simulink model "ERMF_main"  (R2015a)
settings: Solver=ode45  StartTime=0.0  StopTime=10.0  RelTol=1e-3
undefined symbols (not defined in the file or in its folder): EOM
libraries: aerolibutil x4, AERO_lib x1, ATM_lib x1, aerolib6dof2 x1, MOT_lib x1
settings Model: Creator=Andrew  LastModifiedBy=Andrew

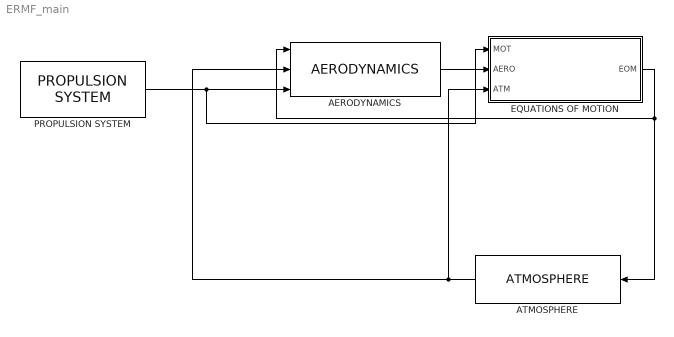
== system ERMF_main ==
  AERODYNAMICS : AERO_lib/AERODYNAMICS
  ATMOSPHERE : ATM_lib/ATMOSPHERE
  EQUATIONS OF MOTION : Subsystem  AncestorBlock=EOM_lib/EQUATIONS OF MOTION
  PROPULSION SYSTEM : MOT_lib/PROPULSION SYSTEM
  wires:
  ATMOSPHERE/1 -> EQUATIONS OF MOTION/3(ATM), AERODYNAMICS/2
  AERODYNAMICS/1 -> EQUATIONS OF MOTION/2(AERO)
  PROPULSION SYSTEM/1 -> EQUATIONS OF MOTION/1(MOT), AERODYNAMICS/3
  EQUATIONS OF MOTION/1(EOM) -> ATMOSPHERE/1, AERODYNAMICS/1

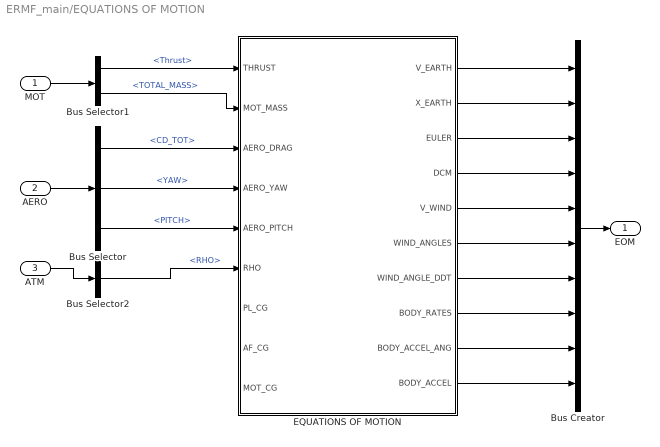
== system ERMF_main/EQUATIONS OF MOTION ==
  MOT : Inport
  AERO : Inport  Port=2
  ATM : Inport  Port=3
  Bus Creator : BusCreator  Inputs=10
  Bus Selector : BusSelector  OutputSignals=AERO_PROP.CD_TOT,VEHICLE.AIRFRAME.YAW,VEHICLE.AIRFRAME.PITCH
  Bus Selector1 : BusSelector  OutputSignals=Thrust,TOTAL_MASS
  Bus Selector2 : BusSelector  OutputSignals=RHO
  EQUATIONS OF MOTION : Subsystem
  EOM : Outport
  wires:
  AERO/1 -> Bus Selector/1
  Bus Selector/1 -> EQUATIONS OF MOTION/3(AERO_DRAG)  "<CD_TOT>"
  Bus Selector/3 -> EQUATIONS OF MOTION/5(AERO_PITCH)  "<PITCH>"
  Bus Selector/2 -> EQUATIONS OF MOTION/4(AERO_YAW)  "<YAW>"
  MOT/1 -> Bus Selector1/1
  Bus Selector1/1 -> EQUATIONS OF MOTION/1(THRUST)  "<Thrust>"
  Bus Selector1/2 -> EQUATIONS OF MOTION/2(MOT_MASS)  "<TOTAL_MASS>"
  ATM/1 -> Bus Selector2/1
  Bus Selector2/1 -> EQUATIONS OF MOTION/6(RHO)  "<RHO>"
  Bus Creator/1 -> EOM/1
  EQUATIONS OF MOTION/4(DCM) -> Bus Creator/4
  EQUATIONS OF MOTION/5(V_WIND) -> Bus Creator/5
  EQUATIONS OF MOTION/2(X_EARTH) -> Bus Creator/2
  EQUATIONS OF MOTION/3(EULER) -> Bus Creator/3
  EQUATIONS OF MOTION/1(V_EARTH) -> Bus Creator/1
  EQUATIONS OF MOTION/9(BODY_ACCEL_ANG) -> Bus Creator/9
  EQUATIONS OF MOTION/10(BODY_ACCEL) -> Bus Creator/10
  EQUATIONS OF MOTION/6(WIND_ANGLES) -> Bus Creator/6
  EQUATIONS OF MOTION/8(BODY_RATES) -> Bus Creator/8
  EQUATIONS OF MOTION/7(WIND_ANGLE_DDT) -> Bus Creator/7

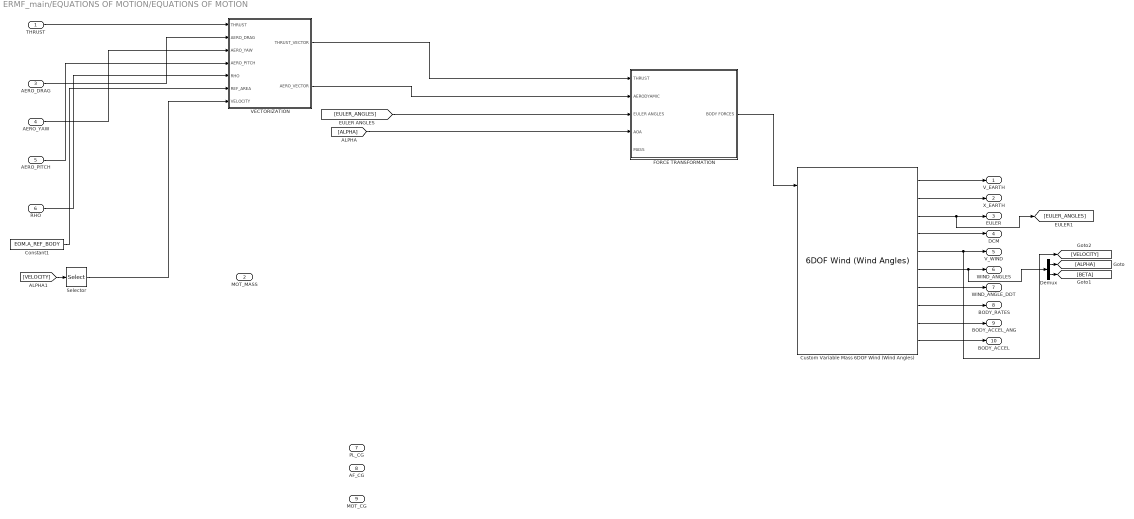
== system ERMF_main/EQUATIONS OF MOTION/EQUATIONS OF MOTION ==
  THRUST : Inport
  MOT_MASS : Inport  Port=2
  AERO_DRAG : Inport  Port=3
  AERO_YAW : Inport  Port=4
  AERO_PITCH : Inport  Port=5
  RHO : Inport  Port=6
  PL_CG : Inport  Port=7
  AF_CG : Inport  Port=8
  MOT_CG : Inport  Port=9
  Constant1 : Constant  Value=EOM.A_REF_BODY
  Custom Variable Mass 6DOF Wind (Wind Angles) : aerolib6dof2/6DOF Wind (Wind Angles)  units=Metric (MKS)  mtype=Custom Variable  rep=Wind Angles  xme_0=[0 0 0]  Vm_0=[0 0 0]  wind_0=[0 0 0]  pm_0=[0 0 0]  mass_0=1.0  mass_e=0.5  mass_f=2.0  inertia=eye(3)  inertia_e=eye(3)  inertia_f=2*eye(3)  vre_flag=off
  Demux : Demux  Outputs=2
  FORCE TRANSFORMATION : Subsystem
  Selector : Selector  InputPortWidth=3  Indices=[1]
  VECTORIZATION : Subsystem
  V_EARTH : Outport
  X_EARTH : Outport  Port=2
  EULER : Outport  Port=3
  DCM : Outport  Port=4
  V_WIND : Outport  Port=5
  WIND_ANGLES : Outport  Port=6
  WIND_ANGLE_DDT : Outport  Port=7
  BODY_RATES : Outport  Port=8
  BODY_ACCEL_ANG : Outport  Port=9
  BODY_ACCEL : Outport  Port=10
  wires:
  [EULER_ANGLES] -> FORCE TRANSFORMATION/3(EULER ANGLES)
  FORCE TRANSFORMATION/1(BODY FORCES) -> Custom Variable Mass 6DOF Wind (Wind Angles)/1
  [ALPHA] -> FORCE TRANSFORMATION/4(AOA)
  Demux/1 -> [ALPHA]
  Demux/2 -> [BETA]
  Custom Variable Mass 6DOF Wind (Wind Angles)/1 -> V_EARTH/1
  Custom Variable Mass 6DOF Wind (Wind Angles)/2 -> X_EARTH/1
  Custom Variable Mass 6DOF Wind (Wind Angles)/3 -> [EULER_ANGLES], EULER/1
  Custom Variable Mass 6DOF Wind (Wind Angles)/4 -> DCM/1
  Custom Variable Mass 6DOF Wind (Wind Angles)/5 -> [VELOCITY], V_WIND/1
  Custom Variable Mass 6DOF Wind (Wind Angles)/6 -> Demux/1, WIND_ANGLES/1
  Custom Variable Mass 6DOF Wind (Wind Angles)/7 -> WIND_ANGLE_DDT/1
  Custom Variable Mass 6DOF Wind (Wind Angles)/8 -> BODY_RATES/1
  Custom Variable Mass 6DOF Wind (Wind Angles)/9 -> BODY_ACCEL_ANG/1
  Custom Variable Mass 6DOF Wind (Wind Angles)/10 -> BODY_ACCEL/1
  THRUST/1 -> VECTORIZATION/1(THRUST)
  AERO_DRAG/1 -> VECTORIZATION/2(AERO_DRAG)
  AERO_YAW/1 -> VECTORIZATION/3(AERO_YAW)
  AERO_PITCH/1 -> VECTORIZATION/4(AERO_PITCH)
  RHO/1 -> VECTORIZATION/5(RHO)
  Constant1/1 -> VECTORIZATION/6(REF_AREA)
  VECTORIZATION/1(THRUST_VECTOR) -> FORCE TRANSFORMATION/1(THRUST)
  VECTORIZATION/2(AERO_VECTOR) -> FORCE TRANSFORMATION/2(AERODYAMIC)
  [VELOCITY] -> Selector/1
  Selector/1 -> VECTORIZATION/7(VELOCITY)

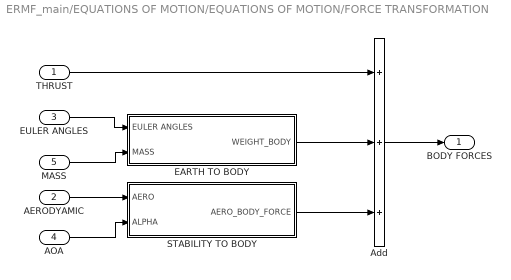
== system ERMF_main/EQUATIONS OF MOTION/EQUATIONS OF MOTION/FORCE TRANSFORMATION ==
  THRUST : Inport
  AERODYAMIC : Inport  Port=2
  EULER ANGLES : Inport  Port=3
  AOA : Inport  Port=4
  MASS : Inport  Port=5
  Add : Sum  Inputs=+++
  EARTH TO BODY : Subsystem
  STABILITY TO BODY : Subsystem
  BODY FORCES : Outport
  wires:
  AOA/1 -> STABILITY TO BODY/2(ALPHA)
  Add/1 -> BODY FORCES/1
  THRUST/1 -> Add/1
  STABILITY TO BODY/1(AERO_BODY_FORCE) -> Add/3
  AERODYAMIC/1 -> STABILITY TO BODY/1(AERO)
  EARTH TO BODY/1(WEIGHT_BODY) -> Add/2
  MASS/1 -> EARTH TO BODY/2(MASS)
  EULER ANGLES/1 -> EARTH TO BODY/1(EULER ANGLES)

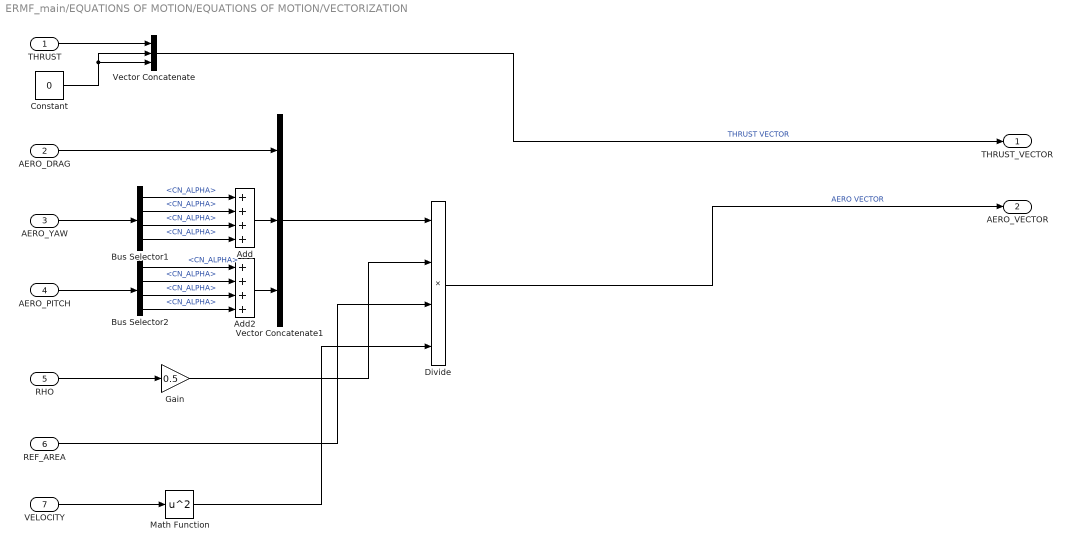
== system ERMF_main/EQUATIONS OF MOTION/EQUATIONS OF MOTION/VECTORIZATION ==
  THRUST : Inport
  AERO_DRAG : Inport  Port=2
  AERO_YAW : Inport  Port=3
  AERO_PITCH : Inport  Port=4
  RHO : Inport  Port=5
  REF_AREA : Inport  Port=6
  VELOCITY : Inport  Port=7
  Add : Sum  Inputs=++++
  Add2 : Sum  Inputs=++++
  Bus Selector1 : BusSelector  OutputSignals=NC.CN_ALPHA,AF_1.CN_ALPHA,AF_2.CN_ALPHA,FIN.CN_ALPHA
  Bus Selector2 : BusSelector  OutputSignals=NC.CN_ALPHA,AF_1.CN_ALPHA,AF_2.CN_ALPHA,FIN.CN_ALPHA
  Constant : Constant  Value=0
  Divide : Product  Inputs=****
  Gain : Gain  Gain=0.5
  Math Function : Math  Operator=square  SaturateOnIntegerOverflow=on
  Vector Concatenate : Concatenate  NumInputs=3
  Vector Concatenate1 : Concatenate  NumInputs=3
  THRUST_VECTOR : Outport
  AERO_VECTOR : Outport  Port=2
  wires:
  Bus Selector2/2 -> Add2/2  "<CN_ALPHA>"
  Bus Selector2/3 -> Add2/3  "<CN_ALPHA>"
  Divide/1 -> AERO_VECTOR/1  "AERO VECTOR"
  THRUST/1 -> Vector Concatenate/1
  Gain/1 -> Divide/2
  Math Function/1 -> Divide/4
  AERO_DRAG/1 -> Vector Concatenate1/1
  AERO_PITCH/1 -> Bus Selector2/1
  AERO_YAW/1 -> Bus Selector1/1
  Vector Concatenate1/1 -> Divide/1
  VELOCITY/1 -> Math Function/1
  Add/1 -> Vector Concatenate1/2
  REF_AREA/1 -> Divide/3
  Bus Selector1/3 -> Add/3  "<CN_ALPHA>"
  Bus Selector2/1 -> Add2/1  "<CN_ALPHA>"
  Add2/1 -> Vector Concatenate1/3
  Bus Selector2/4 -> Add2/4  "<CN_ALPHA>"
  Bus Selector1/4 -> Add/4  "<CN_ALPHA>"
  Bus Selector1/2 -> Add/2  "<CN_ALPHA>"
  Bus Selector1/1 -> Add/1  "<CN_ALPHA>"
  Vector Concatenate/1 -> THRUST_VECTOR/1  "THRUST VECTOR"
  RHO/1 -> Gain/1
  Constant/1 -> Vector Concatenate/2, Vector Concatenate/3

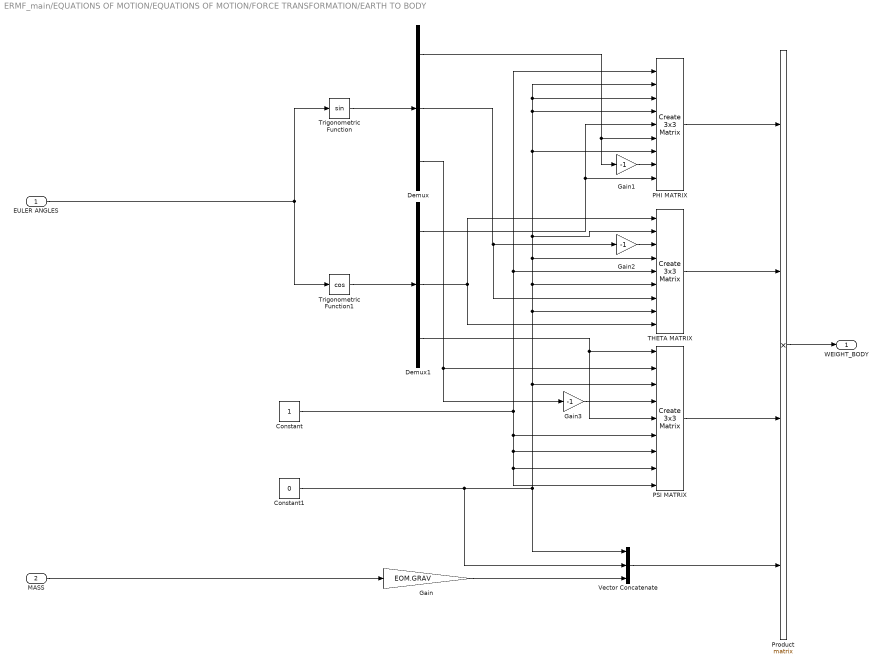
== system ERMF_main/EQUATIONS OF MOTION/EQUATIONS OF MOTION/FORCE TRANSFORMATION/EARTH TO BODY ==
  EULER ANGLES : Inport
  MASS : Inport  Port=2
  Constant : Constant
  Constant1 : Constant  Value=0
  Demux : Demux  Outputs=3
  Demux1 : Demux  Outputs=3
  Gain : Gain  Gain=EOM.GRAV
  Gain1 : Gain  Gain=-1
  Gain2 : Gain  Gain=-1
  Gain3 : Gain  Gain=-1
  "PHI MATRIX " : aerolibutil/Create 3x3 Matrix
  PSI MATRIX : aerolibutil/Create 3x3 Matrix
  Product : Product  Inputs=4  Multiplication=Matrix(*)
  THETA MATRIX : aerolibutil/Create 3x3 Matrix
  Trigonometric Function : Trigonometry
  Trigonometric Function1 : Trigonometry  Operator=cos
  Vector Concatenate : Concatenate  NumInputs=3
  WEIGHT_BODY : Outport
  wires:
  Constant/1 -> THETA MATRIX/5, "PHI MATRIX "/1, PSI MATRIX/6, PSI MATRIX/9, PSI MATRIX/8, PSI MATRIX/7
  Gain1/1 -> "PHI MATRIX "/8
  Gain2/1 -> THETA MATRIX/3
  EULER ANGLES/1 -> Trigonometric Function1/1, Trigonometric Function/1
  Demux1/2 -> THETA MATRIX/9, THETA MATRIX/1
  Demux/2 -> Gain2/1, THETA MATRIX/7
  Trigonometric Function/1 -> Demux/1
  Demux1/1 -> "PHI MATRIX "/9, "PHI MATRIX "/5
  Trigonometric Function1/1 -> Demux1/1
  Constant1/1 -> "PHI MATRIX "/2, "PHI MATRIX "/3, "PHI MATRIX "/4, "PHI MATRIX "/7, THETA MATRIX/2, THETA MATRIX/4, THETA MATRIX/6, THETA MATRIX/8, PSI MATRIX/3, Vector Concatenate/1, Vector Concatenate/2
  Gain/1 -> Vector Concatenate/3
  Demux/1 -> "PHI MATRIX "/6, Gain1/1
  MASS/1 -> Gain/1
  "PHI MATRIX "/1 -> Product/1
  THETA MATRIX/1 -> Product/2
  PSI MATRIX/1 -> Product/3
  Vector Concatenate/1 -> Product/4
  Demux1/3 -> PSI MATRIX/1, PSI MATRIX/5
  Demux/3 -> Gain3/1, PSI MATRIX/2
  Gain3/1 -> PSI MATRIX/4
  Product/1 -> WEIGHT_BODY/1

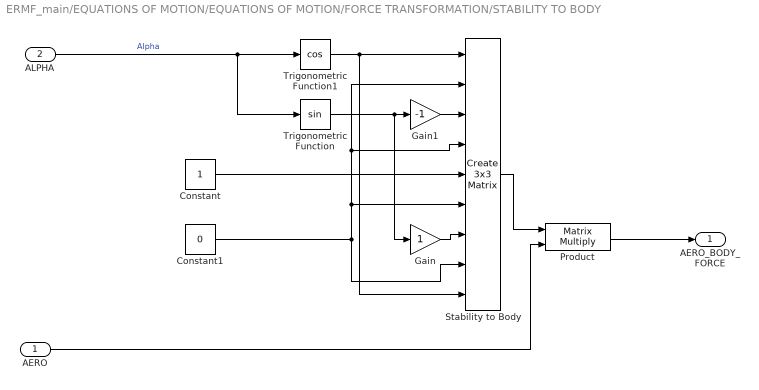
== system ERMF_main/EQUATIONS OF MOTION/EQUATIONS OF MOTION/FORCE TRANSFORMATION/STABILITY TO BODY ==
  AERO : Inport
  ALPHA : Inport  Port=2
  Constant : Constant
  Constant1 : Constant  Value=0
  Gain : Gain
  Gain1 : Gain  Gain=-1
  Product : Product  Multiplication=Matrix(*)
  Stability to Body : aerolibutil/Create 3x3 Matrix
  Trigonometric Function : Trigonometry
  Trigonometric Function1 : Trigonometry  Operator=cos
  AERO_BODY_FORCE : Outport
  wires:
  ALPHA/1 -> Trigonometric Function1/1, Trigonometric Function/1  "Alpha"
  Stability to Body/1 -> Product/1
  Constant/1 -> Stability to Body/5
  Trigonometric Function/1 -> Gain1/1, Gain/1
  Gain1/1 -> Stability to Body/3
  Constant1/1 -> Stability to Body/2, Stability to Body/4, Stability to Body/6, Stability to Body/8
  Product/1 -> AERO_BODY_FORCE/1
  AERO/1 -> Product/2
  Trigonometric Function1/1 -> Stability to Body/1, Stability to Body/9
  Gain/1 -> Stability to Body/7
